simulink model "Udan_SOC"  (R2017b)
settings: Solver=FixedStepAuto  StartTime=0.0  StopTime=1000  FixedStep=0.1  RelTol=1e-3
values from neighbouring files (symbols this model uses):
  DenominatorOfIntegratorFactor = 100.0    [SOC_Stateflow.sldd]
  SOC_CalcSohLKT = 1.0    [SOC_Stateflow.sldd]
  SOC_CalcSOHTempLimit = 70.0    [SOC_Stateflow.sldd]
  SOC_CapPerCycle = 100.0    [SOC_Stateflow.sldd]
  SOC_CapTemp_HLimit = 200.0    [SOC_Stateflow.sldd]
  SOC_CapTemp_LLimit = 0.0    [SOC_Stateflow.sldd]
  Soc_ConfigInfo = 0    [SOC_Stateflow.sldd]
  SOC_DchgEndCalib = 0.0    [SOC_Stateflow.sldd]
  SOC_DiffVoltMin = 10.0    [SOC_Stateflow.sldd]
  SOC_DSOCJumpMax = 500.0    [SOC_Stateflow.sldd]
  SOC_EfficientHighLimit = 250.0    [SOC_Stateflow.sldd]
  SOC_EfficientLowLimit = 40.0    [SOC_Stateflow.sldd]
  SOC_EmptyAus = 0.0    [SOC_Stateflow.sldd]
  SOC_EnableOcv = 1.0    [SOC_Stateflow.sldd]
  SOC_END_CALIB_STATE : value not decoded    [SOC_Stateflow.sldd]
  SOC_HighRealSoc = 95.0    [SOC_Stateflow.sldd]
  SOC_LKTSohCycles = 0.0 1.0 10.0 20.0 30.0 40.0 50.0 60.0 70.0 80.0 90.0 100.0 110.0 120.0 130.0 140.0 150.0 160.0 170.0 180.0 190.0 200.0 210.0 220.0 230.0 240.0 250.0 260.0 270.0 280.0 290.0 300.0 310.0 320.0 330.0 340.0 350.0 360.0 370.0 380.0 390.0 400.0 410.0 420.0 430.0 440.0 450.0 460.0 470.0 480.0 490.0 500.0 510.0 520.0 530.0 540.0 550.0 560.0 570.0 580.0 590.0 600.0 610.0 620.0 630.0 640.0 650.0 660.0 670.0    [SOC_Stateflow.sldd]
  SOC_LKTSohTable = 1000.0 991.0 989.0 992.0 993.0 995.0 994.0 993.0 1000.0 997.0 1002.0 1000.0 992.0 1000.0 989.0 992.0 989.0 994.0 989.0 993.0 994.0 994.0 994.0 993.0 991.0 991.0 992.0 993.0 991.0 985.0 985.0 985.0 979.0 975.0 978.0 984.0 982.0 974.0 975.0 972.0 972.0 975.0 977.0 977.0 974.0 971.0 973.0 971.0 966.0 968.0 965.0 959.0 957.0 956.0 957.0 954.0 955.0 951.0 954.0 951.0 942.0 942.0 940.0 942.0 947.0 949.0    [SOC_Stateflow.sldd]
  SOC_LowRealSoc = 5.0    [SOC_Stateflow.sldd]
  SOC_NominalCap_AmS = 576000000.0    [SOC_Stateflow.sldd]
  SOC_NominalVol = 4000.0    [SOC_Stateflow.sldd]
  SOC_OCVTemp_HLimit = 106.0    [SOC_Stateflow.sldd]
  SOC_OCVTemp_LLimit = 29.0    [SOC_Stateflow.sldd]
  SOC_ShortCalibDSoc = 1.0    [SOC_Stateflow.sldd]
  SOC_SOCResolution = 10000.0    [SOC_Stateflow.sldd]
  SOC_SohCalcCapPercent = 8.0    [SOC_Stateflow.sldd]
  SOC_SohCalcHighLimit = 60.0    [SOC_Stateflow.sldd]
  SOC_SohCalcLowLimit = 10.0    [SOC_Stateflow.sldd]
  SOC_SohCalcMidLimit = 30.0    [SOC_Stateflow.sldd]
  SOC_SOHResolution = 1000.0    [SOC_Stateflow.sldd]
  SOC_State = <binary blob, 1163 chars, not shown>    [SOC_Stateflow.sldd]
  SOC_TempCap_CapBuffer : value not decoded    [SOC_Stateflow.sldd]
  SOC_TempCap_TempBuffer : value not decoded    [SOC_Stateflow.sldd]
  SocOcvCalib_ConfigInfo = 0.0    [SOC_Stateflow.sldd]
  SocOcvCalib_SocBuffer1 : value not decoded    [SOC_Stateflow.sldd]
  SocOcvCalib_TempBuffer : value not decoded    [SOC_Stateflow.sldd]
  SocOcvCalib_VoltageBuffer1 = 3300.0 3303.0 3305.0 3307.0 3310.0 3311.0 3313.0 3314.0 3316.0 3317.0 3319.0 3320.0 3322.0 3323.0 3325.0 3322.0 3323.0 3325.0 3310.0 3313.0 3315.0 3317.0 3320.0 3321.0 3323.0 3324.0 3326.0 3327.0 3329.0 3330.0 3332.0 3333.0 3335.0 3332.0 3333.0 3335.0 3320.0 3323.0 3325.0 3327.0 3330.0 3331.0 3333.0 3334.0 3336.0 3337.0 3339.0 3340.0 3342.0 3343.0 3345.0 3342.0 3343.0 3345.0 3330.0 3333.0 3335.0 3    [SOC_Stateflow.sldd]
  SOHCalibCycle = 10.0    [SOC_Stateflow.sldd]
undefined symbols (not defined in the file or in its folder): DatetimeM_GetReturnType, ParameterM_EeepParaIndexType, Soc_CumuLativeTypeType, SOC_EgthTempChgValue, Soc_EnergyBuffer, SOC_FithTempChgValue, SOC_FstSlowTempChgValue, SOC_FstTempChgValue, SOC_FthTempChgValue, SOC_MaxCap_AmS, SOC_SethTempChgValue, SOC_SixTempChgValue, SOC_SndSlowTempChgValue, SOC_SndTempChgValue, SOC_TrdSlowTempChgValue, SOC_TrdTempChgValue, SocDiagCalib_NoCalibReasonType
libraries: simulink x138, hdlsllib x24, dspindex x4
(part 5 of 10)

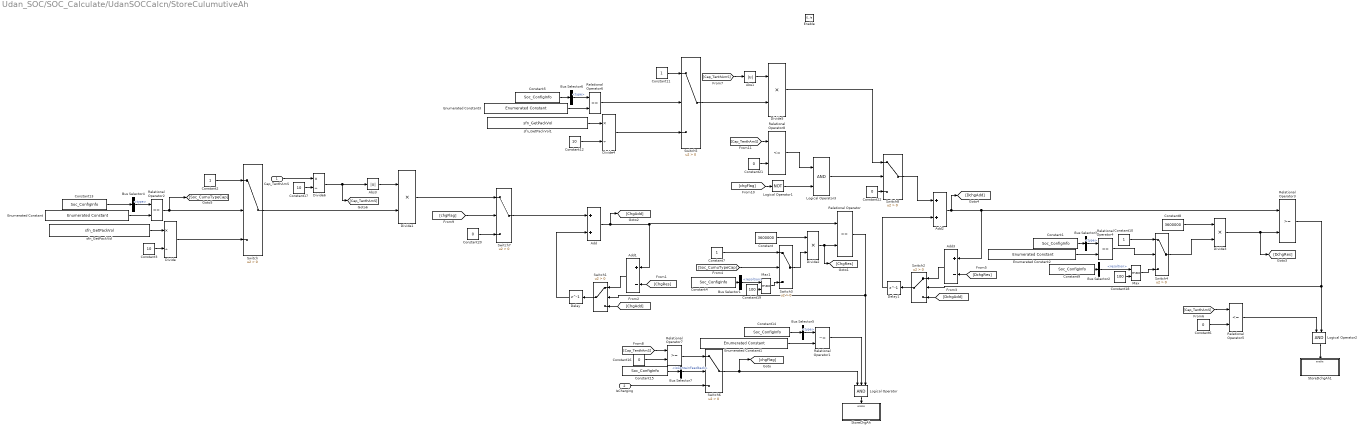
== system Udan_SOC/SOC_Calculate/UdanSOCCalcn/StoreCulumutiveAh ==
  Cap_TenthAmS : Inport
  IsCharging : Inport  Port=2
  Enable : EnablePort
  Abs1 : Abs
  Abs3 : Abs
  Add : Sum  OutDataTypeStr=uint32
  Add1 : Sum  Inputs=+-  OutDataTypeStr=int32
  Add2 : Sum  OutDataTypeStr=uint32
  Add3 : Sum  Inputs=+-  OutDataTypeStr=int32
  Bus Selector1 : BusSelector  OutputSignals=ChgCumuInfo.resoltion
  Bus Selector2 : BusSelector  OutputSignals=DchgCumuInfo.resoltion
  Bus Selector3 : BusSelector  OutputSignals=DchgCumuInfo.type
  Bus Selector4 : BusSelector  OutputSignals=ChgCumuInfo.type
  Bus Selector5 : BusSelector  OutputSignals=ChgCumuInfo.type
  Bus Selector6 : BusSelector  OutputSignals=DchgCumuInfo.type
  Bus Selector7 : BusSelector  OutputSignals=ChgCumuInfo.isContainFeedback
  Constant : Constant  Value=3600000  OutDataTypeStr=uint32
  Constant{1,4..5,9,13..15} (7 alike) : Constant  Value=Soc_ConfigInfo  OutDataTypeStr=Bus: Soc_ConfigInfoType
  Constant{2,7,10..11} (4 alike) : Constant  OutDataTypeStr=uint16
  Constant12 : Constant  Value=10  OutDataTypeStr=uint8
  Constant16 : Constant  Value=0  OutDataTypeStr=uint8
  Constant17 : Constant  Value=10  OutDataTypeStr=uint8
  Constant18 : Constant  Value=100  OutDataTypeStr=uint16
  Constant19 : Constant  Value=100  OutDataTypeStr=uint16
  Constant20 : Constant  Value=0  OutDataTypeStr=uint32
  Constant21 : Constant  Value=0  OutDataTypeStr=int8
  Constant22 : Constant  Value=0  OutDataTypeStr=uint32
  Constant3 : Constant  Value=10  OutDataTypeStr=uint8
  Constant6 : Constant  Value=0  OutDataTypeStr=uint8
  Constant8 : Constant  Value=3600000  OutDataTypeStr=uint32
  Delay : Delay  DelayLength=1  InitialCondition=0
  Delay1 : Delay  DelayLength=1  InitialCondition=0
  Divide : Product  Inputs=*/  OutDataTypeStr=uint16
  Divide{1..3,5} (4 alike) : Product  Inputs=**  OutDataTypeStr=uint32
  Divide4 : Product  Inputs=*/  OutDataTypeStr=uint16
  Divide6 : Product  Inputs=*/  OutDataTypeStr=int32
  Enumerated Constant : simulink/Sources/Enumerated Constant  OutDataTypeStr=Enum: Soc_CumuLativeTypeType  Value=Soc_CumuLativeTypeType.Soc_CumuTypeCap  SampleTime=inf
      settings: SourceProductName=Simulink
  Enumerated Constant1 : simulink/Sources/Enumerated Constant  OutDataTypeStr=Enum: Soc_CumuLativeTypeType  Value=Soc_CumuLativeTypeType.Soc_CumuTypeNone  SampleTime=inf
      settings: SourceProductName=Simulink
  Enumerated Constant2 : simulink/Sources/Enumerated Constant  OutDataTypeStr=Enum: Soc_CumuLativeTypeType  Value=Soc_CumuLativeTypeType.Soc_CumuTypeCap  SampleTime=inf
      settings: SourceProductName=Simulink
  Enumerated Constant3 : simulink/Sources/Enumerated Constant  OutDataTypeStr=Enum: Soc_CumuLativeTypeType  Value=Soc_CumuLativeTypeType.Soc_CumuTypeCap  SampleTime=inf
      settings: SourceProductName=Simulink
  Logical Operator : Logic  Inputs=3  AllPortsSameDT=off  OutDataTypeStr=boolean
  Logical Operator1 : Logic  Operator=NOT  AllPortsSameDT=off  OutDataTypeStr=boolean
  Logical Operator2 : Logic  AllPortsSameDT=off  OutDataTypeStr=boolean
  Logical Operator3 : Logic  AllPortsSameDT=off  OutDataTypeStr=boolean
  Max : MinMax  Function=max  Inputs=2
  Max1 : MinMax  Function=max  Inputs=2
  Relational Operator : RelationalOperator  OutDataTypeStr=boolean  RndMeth=Simplest
  Relational Operator1 : RelationalOperator  Operator=~=  OutDataTypeStr=boolean  RndMeth=Simplest
  Relational Operator2 : RelationalOperator  Operator===  OutDataTypeStr=boolean  RndMeth=Simplest
  Relational Operator3 : RelationalOperator  OutDataTypeStr=boolean  RndMeth=Simplest
  Relational Operator4 : RelationalOperator  Operator===  OutDataTypeStr=boolean  RndMeth=Simplest
  Relational Operator5 : RelationalOperator  Operator=<=  OutDataTypeStr=boolean  RndMeth=Simplest
  Relational Operator6 : RelationalOperator  Operator===  OutDataTypeStr=boolean  RndMeth=Simplest
  Relational Operator7 : RelationalOperator  OutDataTypeStr=boolean  RndMeth=Simplest
  Relational Operator8 : RelationalOperator  Operator=<=  OutDataTypeStr=boolean  RndMeth=Simplest
  StoreChgAh : Subsystem  TreatAsAtomicUnit=on
  StoreDchgAh1 : Subsystem  TreatAsAtomicUnit=on
  Switch{,1..2,5..8} (7 alike) : Switch  Criteria=u2 > Threshold
  Switch3 : Switch  Criteria=u2 > Threshold  OutDataTypeStr=uint16
  Switch4 : Switch  Criteria=u2 > Threshold  OutDataTypeStr=uint16
  sfn_GetPackVol : S-Function  FunctionName=sfn_GetPackVol  SFunctionDeploymentMode=off  EnableBusSupport=off  mask(Legacy Function){SFunctionSpec=uint16 y1=Statistic_GetBcu100mvTotalVoltage(void), ShowSpec=on}
      mask prompts: ShowSpec "Display function specification"
      mask help:
      | This block allows you to call the legacy functions specified by the following Legacy Code Tool definition:
      | def.SFunctionName = 'sfn_GetPackVol';
      | def.OutputFcnSpec = 'uint16 y1=Statistic_GetBcu100mvTotalVoltage(void)';
      | def.HeaderFiles = {'Statistic.h'};
      mask Help: <p>This block was generated automatically by the Legacy Code Tool. For detailed help on this tool, call<a href="matlab:legacy_code('help')"> legacy_code('help')</a>.</p>
      mask Callback ShowSpec:
      | if strcmp(get_param(gcbh, 'ShowSpec'), 'on')
      |   set_param(gcbh, 'MaskDisplay', sprintf('fprintf(''%s'');', get_param(gcbh, 'SFunctionSpec')));
      | else
      |   set_param(gcbh, 'MaskDisplay', sprintf('fprintf(''%s'');', get_param(gcbh, 'FunctionName')));
      | end
      mask Display: fprintf('uint16 y1=Statistic_GetBcu100mvTotalVoltage(void)');
  sfn_GetPackVol1 : S-Function  FunctionName=sfn_GetPackVol  SFunctionDeploymentMode=off  EnableBusSupport=off  mask(Legacy Function){SFunctionSpec=uint16 y1=Statistic_GetBcu100mvTotalVoltage(void), ShowSpec=on}
      mask prompts: ShowSpec "Display function specification"
      mask help:
      | This block allows you to call the legacy functions specified by the following Legacy Code Tool definition:
      | def.SFunctionName = 'sfn_GetPackVol';
      | def.OutputFcnSpec = 'uint16 y1=Statistic_GetBcu100mvTotalVoltage(void)';
      | def.HeaderFiles = {'Statistic.h'};
      mask Help: <p>This block was generated automatically by the Legacy Code Tool. For detailed help on this tool, call<a href="matlab:legacy_code('help')"> legacy_code('help')</a>.</p>
      mask Callback ShowSpec:
      | if strcmp(get_param(gcbh, 'ShowSpec'), 'on')
      |   set_param(gcbh, 'MaskDisplay', sprintf('fprintf(''%s'');', get_param(gcbh, 'SFunctionSpec')));
      | else
      |   set_param(gcbh, 'MaskDisplay', sprintf('fprintf(''%s'');', get_param(gcbh, 'FunctionName')));
      | end
      mask Display: fprintf('uint16 y1=Statistic_GetBcu100mvTotalVoltage(void)');
  wires:
  Abs3/1 -> Divide1/1
  Switch7/1 -> Add/1
  Bus Selector3/1 -> Relational Operator4/1  "<type>"
  Constant1/1 -> Bus Selector3/1
  Enumerated Constant2/1 -> Relational Operator4/2
  Constant14/1 -> Bus Selector5/1
  Relational Operator1/1 -> Logical Operator/2
  Enumerated Constant1/1 -> Relational Operator1/2
  Bus Selector5/1 -> Relational Operator1/1  "<type>"
  Add2/1 -> [DchgAdd], Add3/1, Relational Operator3/1
  Delay1/1 -> Add2/2
  [DchgRes] -> Add3/2
  Switch2/1 -> Delay1/1
  [DchgAdd] -> Switch2/3
  Add3/1 -> Switch2/1
  Delay/1 -> Add/2
  [ChgAdd] -> Switch1/3
  Add1/1 -> Switch1/1
  [ChgRes] -> Add1/2
  Relational Operator/1 -> Logical Operator/3, Switch1/2
  Relational Operator3/1 -> Logical Operator2/2, Switch2/2
  Divide3/1 -> Relational Operator3/2, [DchgRes]
  Divide2/1 -> [ChgRes], Relational Operator/2
  Constant4/1 -> Bus Selector1/1
  Bus Selector1/1 -> Max1/1  "<resoltion>"
  IsCharging/1 -> Switch6/3
  Switch/1 -> Divide1/2
  Divide6/1 -> [Cap_TenthAmS], Abs3/1
  Divide/1 -> Switch/3
  Constant3/1 -> Divide/2
  sfn_GetPackVol/1 -> Divide/1
  Constant2/1 -> Switch/1
  Relational Operator2/1 -> Switch/2, [Soc_CumuTypeCap]
  Enumerated Constant/1 -> Relational Operator2/2
  Constant13/1 -> Bus Selector4/1
  Bus Selector4/1 -> Relational Operator2/1  "<type>"
  Logical Operator2/1 -> StoreDchgAh1/Enable
  Logical Operator/1 -> StoreChgAh/Enable
  Constant/1 -> Divide2/1
  Add/1 -> Add1/1, Relational Operator/1, [ChgAdd]
  Switch1/1 -> Delay/1
  [Soc_CumuTypeCap] -> Switch3/2
  Constant7/1 -> Switch3/1
  Switch3/1 -> Divide2/2
  Relational Operator5/1 -> Logical Operator2/1
  [Cap_TenthAmS] -> Relational Operator5/1
  Constant6/1 -> Relational Operator5/2
  Switch4/1 -> Divide3/2
  Bus Selector2/1 -> Max/1  "<resoltion>"
  Constant9/1 -> Bus Selector2/1
  Constant8/1 -> Divide3/1
  Relational Operator4/1 -> Switch4/2
  Constant10/1 -> Switch4/1
  Constant11/1 -> Switch5/1
  Relational Operator6/1 -> Switch5/2
  Constant5/1 -> Bus Selector6/1
  Enumerated Constant3/1 -> Relational Operator6/2
  Bus Selector6/1 -> Relational Operator6/1  "<type>"
  Constant12/1 -> Divide4/2
  Divide4/1 -> Switch5/3
  sfn_GetPackVol1/1 -> Divide4/1
  [Cap_TenthAmS] -> Abs1/1
  Switch5/1 -> Divide5/2
  Divide5/1 -> Switch8/1
  Abs1/1 -> Divide5/1
  Constant15/1 -> Bus Selector7/1
  Constant16/1 -> Relational Operator7/2
  [Cap_TenthAmS] -> Relational Operator7/1
  Bus Selector7/1 -> Switch6/2  "<isContainFeedback>"
  Relational Operator7/1 -> Switch6/1
  Switch6/1 -> [chgFlag], Logical Operator/1
  Cap_TenthAmS/1 -> Divide6/1
  Constant17/1 -> Divide6/2
  Constant18/1 -> Max/2
  Max/1 -> Switch4/3
  Constant19/1 -> Max1/2
  Max1/1 -> Switch3/3
  [chgFlag] -> Switch7/2
  Divide1/1 -> Switch7/1
  Constant20/1 -> Switch7/3
  [chgFlag] -> Logical Operator1/1
  [Cap_TenthAmS] -> Relational Operator8/1
  Constant21/1 -> Relational Operator8/2
  Relational Operator8/1 -> Logical Operator3/1
  Logical Operator1/1 -> Logical Operator3/2
  Logical Operator3/1 -> Switch8/2
  Constant22/1 -> Switch8/3
  Switch8/1 -> Add2/1

== system Udan_SOC/SOC_Calculate/UdanSOCCalcn/StoreDSOC ==
  LastCap : Inport
  SocCalibFlag : Inport  Port=2  OutDataTypeStr=uint8  PortDimensions=[1]
  OcvCmd : Inport  Port=3
  Abs : Abs
  Bus Selector : BusSelector  OutputSignals=soc
  Constant1 : Constant  OutDataTypeStr=uint8
  Constant6 : Constant  Value=50  OutDataTypeStr=uint8
  Delay1 : Delay  DelayLength=1  InitialCondition=0
  Logical Operator : Logic  AllPortsSameDT=off  OutDataTypeStr=boolean
  Logical Operator1 : Logic  Operator=OR  Inputs=3  AllPortsSameDT=off  OutDataTypeStr=boolean
  Relational Operator1 : RelationalOperator  OutDataTypeStr=boolean  RndMeth=Simplest
  Relational Operator3 : RelationalOperator  OutDataTypeStr=boolean  RndMeth=Simplest
  Subtract : Sum  Inputs=+-  AccumDataTypeStr=int32  OutDataTypeStr=int32
  Switch : Switch  Criteria=u2 > Threshold
  WriteLeftCap : Subsystem  TreatAsAtomicUnit=on
  wires:
  Bus Selector/1 -> Relational Operator1/1, Switch/1, WriteLeftCap/1(DSOC), Subtract/2  "<soc>"
  Relational Operator3/1 -> Logical Operator1/3, Switch/2
  Switch/1 -> Delay1/1
  Delay1/1 -> Switch/3, [WritedCap]
  Abs/1 -> Relational Operator3/1
  Constant6/1 -> Relational Operator3/2
  Subtract/1 -> Abs/1
  [WritedCap] -> Subtract/1
  LastCap/1 -> Bus Selector/1
  Logical Operator/1 -> WriteLeftCap/Enable
  Constant1/1 -> Relational Operator1/2
  Relational Operator1/1 -> Logical Operator/1
  Logical Operator1/1 -> Logical Operator/2
  SocCalibFlag/1 -> Logical Operator1/2
  OcvCmd/1 -> Logical Operator1/1

== system Udan_SOC/SOC_Calculate/UdanSOCCalcn/StoreLeftCap ==
  LastCap : Inport
  OcvCmd : Inport  Port=2
  SocCalibFlag : Inport  Port=3  OutDataTypeStr=uint8  PortDimensions=[1]
  Constant : Constant  Value=SOC_SOCResolution
  Constant1 : Constant  Value=SOC_NominalCap_AmS
  Constant4 : Constant  Value=SOC_NominalCap_AmS
  Constant5 : Constant  Value=1000  OutDataTypeStr=uint32
  Constant6 : Constant  Value=8  OutDataTypeStr=uint32
  Delay1 : Delay  DelayLength=1  InitialCondition=0
  Divide : Product  Inputs=*/*
  Divide1 : Product  Inputs=*/  OutDataTypeStr=uint32
  Logical Operator : Logic  AllPortsSameDT=off  OutDataTypeStr=boolean
  Logical Operator1 : Logic  Operator=OR  Inputs=3  AllPortsSameDT=off  OutDataTypeStr=boolean
  Logical Operator2 : Logic  Operator=NOT  AllPortsSameDT=off  OutDataTypeStr=boolean
  Relational Operator : RelationalOperator  OutDataTypeStr=boolean  RndMeth=Simplest
  Relational Operator1 : RelationalOperator  OutDataTypeStr=boolean  RndMeth=Simplest
  Relational Operator3 : RelationalOperator  OutDataTypeStr=boolean  RndMeth=Simplest
  Subtract : Sum  Inputs=+-  AccumDataTypeStr=uint32  OutDataTypeStr=uint32
  Switch : Switch  Criteria=u2 > Threshold
  Switch1 : Switch  Criteria=u2 > Threshold
  Switch2 : Switch  Criteria=u2 > Threshold
  WriteLeftCap : Subsystem  TreatAsAtomicUnit=on
  wires:
  LastCap/1 -> Switch2/3, Switch1/3, Relational Operator/2, WriteLeftCap/1(cap), Switch/1, Relational Operator1/1
  Relational Operator3/1 -> Logical Operator1/3, Switch/2
  Switch/1 -> Delay1/1
  Delay1/1 -> Switch/3, [WritedCap]
  Subtract/1 -> Relational Operator3/1
  Divide/1 -> Relational Operator3/2
  Constant6/1 -> Divide/3
  Constant5/1 -> Divide/2
  Constant4/1 -> Divide/1
  [WritedCap] -> Relational Operator/1, Switch2/1, Switch1/1
  Constant1/1 -> Divide1/1
  Constant/1 -> Divide1/2
  Divide1/1 -> Relational Operator1/2
  Relational Operator1/1 -> Logical Operator/1
  Logical Operator/1 -> WriteLeftCap/Enable
  Logical Operator1/1 -> Logical Operator/2
  SocCalibFlag/1 -> Logical Operator1/1
  Relational Operator/1 -> Switch1/2, Logical Operator2/1
  Switch1/1 -> Subtract/1
  Logical Operator2/1 -> Switch2/2
  Switch2/1 -> Subtract/2
  OcvCmd/1 -> Logical Operator1/2

== system Udan_SOC/SOC_Calculate/UdanSOCCalcn/StoreSOC ==
  CurrentAmS : Inport
  IsCharging : Inport  Port=2
  Constant : Constant  Value=0  OutDataTypeStr=uint8
  Constant1 : Constant  Value=0  OutDataTypeStr=uint8
  Logical Operator : Logic  Operator=OR  AllPortsSameDT=off  OutDataTypeStr=boolean
  Logical Operator1 : Logic  AllPortsSameDT=off  OutDataTypeStr=boolean
  Logical Operator2 : Logic  Operator=NOT  AllPortsSameDT=off  OutDataTypeStr=boolean
  Relational Operator : RelationalOperator  Operator=<=  OutDataTypeStr=boolean  RndMeth=Simplest
  Relational Operator1 : RelationalOperator  Operator=>  OutDataTypeStr=boolean  RndMeth=Simplest
  Subsystem : Subsystem
  Subsystem1 : Subsystem
  wires:
  Constant/1 -> Relational Operator/2
  Relational Operator/1 -> Logical Operator/1
  Logical Operator/1 -> Subsystem/Enable
  IsCharging/1 -> [IsCharging], Logical Operator/2
  CurrentAmS/1 -> Relational Operator/1, Subsystem/1(CurrentAmS), Subsystem1/1(CurrentAmS), Relational Operator1/1
  Constant1/1 -> Relational Operator1/2
  Relational Operator1/1 -> Logical Operator1/1
  [IsCharging] -> Logical Operator2/1
  Logical Operator2/1 -> Logical Operator1/2
  Logical Operator1/1 -> Subsystem1/Enable

== system Udan_SOC/SOC_Calculate/UdanSOCCalcn/StoreTSOC ==
  LastCap : Inport
  Abs : Abs
  Bus Selector : BusSelector  OutputSignals=soc
  Constant1 : Constant  OutDataTypeStr=uint8
  Constant6 : Constant  Value=100  OutDataTypeStr=uint8
  Delay1 : Delay  DelayLength=1  InitialCondition=0
  Logical Operator : Logic  AllPortsSameDT=off  OutDataTypeStr=boolean
  Logical Operator1 : Logic  Operator=OR  Inputs=1  AllPortsSameDT=off  OutDataTypeStr=boolean
  Relational Operator1 : RelationalOperator  OutDataTypeStr=boolean  RndMeth=Simplest
  Relational Operator3 : RelationalOperator  OutDataTypeStr=boolean  RndMeth=Simplest
  Subtract : Sum  Inputs=+-  AccumDataTypeStr=int32  OutDataTypeStr=int32
  Switch : Switch  Criteria=u2 > Threshold
  WriteLeftCap : Subsystem  TreatAsAtomicUnit=on
  wires:
  Bus Selector/1 -> Relational Operator1/1, Switch/1, WriteLeftCap/1(DSOC), Subtract/2  "<soc>"
  Relational Operator3/1 -> Logical Operator1/1, Switch/2
  Switch/1 -> Delay1/1
  Delay1/1 -> Switch/3, [WritedCap]
  Abs/1 -> Relational Operator3/1
  Constant6/1 -> Relational Operator3/2
  Subtract/1 -> Abs/1
  [WritedCap] -> Subtract/1
  LastCap/1 -> Bus Selector/1
  Logical Operator/1 -> WriteLeftCap/Enable
  Constant1/1 -> Relational Operator1/2
  Relational Operator1/1 -> Logical Operator/1
  Logical Operator1/1 -> Logical Operator/2

== system Udan_SOC/SOC_Calculate/UdanSOCCalcn/Subsystem1 ==
  HighIndex : Inport
  LowIndex : Inport  Port=2
  DefaultValue : Inport  Port=3
  Constant1 : Constant  Value=0  OutDataTypeStr=uint8
  Constant2 : Constant  Value=0  OutDataTypeStr=uint8
  Logical Operator : Logic  AllPortsSameDT=off  OutDataTypeStr=boolean
  Logical Operator1 : Logic  Operator=NOT  AllPortsSameDT=off  OutDataTypeStr=boolean
  Relational Operator : RelationalOperator  Operator===  OutDataTypeStr=boolean  RndMeth=Simplest
  Relational Operator1 : RelationalOperator  Operator===  OutDataTypeStr=boolean  RndMeth=Simplest
  S-Function : S-Function  FunctionName=sfn_NVMRead  SFunctionDeploymentMode=off  EnableBusSupport=off
  S-Function1 : S-Function  FunctionName=sfn_NVMRead  SFunctionDeploymentMode=off  EnableBusSupport=off
  Subsystem : Subsystem
  Switch : Switch  Criteria=u2 > Threshold
  EeepRead32 : Outport
  wires:
  DefaultValue/1 -> Switch/1
  [ReadLowOk] -> Logical Operator/1
  S-Function/2 -> Subsystem/1(HighIndex)
  S-Function/1 -> Relational Operator/1
  S-Function1/2 -> Subsystem/2(LowIndex)
  HighIndex/1 -> S-Function/1
  Constant1/1 -> Relational Operator/2
  Constant2/1 -> Relational Operator1/2
  LowIndex/1 -> S-Function1/1
  Relational Operator/1 -> Logical Operator/2
  Logical Operator/1 -> Logical Operator1/1, Subsystem/Enable
  Relational Operator1/1 -> [ReadLowOk]
  S-Function1/1 -> Relational Operator1/1
  Subsystem/1(soc) -> Switch/3
  Logical Operator1/1 -> Switch/2
  Switch/1 -> EeepRead32/1

== system Udan_SOC/SOC_Calculate/UdanSOCCalcn/WriteOCVTime ==
  RTCTimeOut : Inport
  OCVCmd : Inport  Port=2
  RtcTime : Inport  Port=3
  function : TriggerPort  TriggerType=function-call  VariantControl=Variant
  Constant : Constant  Value=0  OutDataTypeStr=boolean
  Data Store Write : DataStoreWrite  DataStoreName=LargeCurrentFlag
  Enumerated Constant : simulink/Sources/Enumerated Constant  OutDataTypeStr=Enum: ParameterM_EeepParaIndexType  Value=ParameterM_EeepParaIndexType.PARAMETERM_EEEP_OCVSOC_TIME_HIGH_INDEX  SampleTime=inf
      settings: SourceProductName=Simulink
  Enumerated Constant1 : simulink/Sources/Enumerated Constant  OutDataTypeStr=Enum: ParameterM_EeepParaIndexType  Value=ParameterM_EeepParaIndexType.PARAMETERM_EEEP_OCVSOC_TIME_LOW_INDEX  SampleTime=inf
      settings: SourceProductName=Simulink
  Enumerated Constant2 : simulink/Sources/Enumerated Constant  OutDataTypeStr=Enum: SOC_State  Value=SOC_State.SOC_STATE_DCHGSOH  SampleTime=inf
      settings: SourceProductName=Simulink
  Enumerated Constant6 : simulink/Sources/Enumerated Constant  OutDataTypeStr=Enum: SOC_State  Value=SOC_State.SOC_STATE_OCV_LONG  SampleTime=inf
      settings: SourceProductName=Simulink
  Enumerated Constant7 : simulink/Sources/Enumerated Constant  OutDataTypeStr=Enum: SOC_State  Value=SOC_State.SOC_STATE_OCV  SampleTime=inf
      settings: SourceProductName=Simulink
  Logical Operator : Logic  Operator=OR  Inputs=3  AllPortsSameDT=off  OutDataTypeStr=boolean
  Relational Operator1 : RelationalOperator  Operator===  OutDataTypeStr=boolean  RndMeth=Simplest
  Relational Operator10 : RelationalOperator  Operator===  OutDataTypeStr=boolean  RndMeth=Simplest
  Relational Operator11 : RelationalOperator  Operator===  OutDataTypeStr=boolean  RndMeth=Simplest
  Subsystem : Subsystem  mask(EeepWrite_uint32){}
      mask help: EeepWrite_uint32
  Switch8 : Switch  Criteria=u2 > Threshold
  Terminator : Terminator
  SOC_RTCTime : Outport
  wires:
  RtcTime/1 -> Switch8/1
  Enumerated Constant1/1 -> Subsystem/3(LowIndex)
  Enumerated Constant/1 -> Subsystem/2(HighIndex)
  Constant/1 -> Data Store Write/1
  RTCTimeOut/1 -> Switch8/3
  Switch8/1 -> SOC_RTCTime/1, Subsystem/1(data)
  Enumerated Constant6/1 -> Relational Operator11/2
  Enumerated Constant7/1 -> Relational Operator10/2
  Enumerated Constant2/1 -> Relational Operator1/2
  OCVCmd/1 -> Relational Operator1/1, Relational Operator11/1, Relational Operator10/1
  Relational Operator11/1 -> Logical Operator/2
  Relational Operator10/1 -> Logical Operator/1
  Relational Operator1/1 -> Logical Operator/3
  Logical Operator/1 -> Switch8/2
  Subsystem/1(WriteResult) -> Terminator/1

== system Udan_SOC/SOC_Calculate/UdanSOCCalcn/WriteSOH ==
  SOH : Inport
  Enable : EnablePort
  Data Type Conversion : DataTypeConversion  OutDataTypeStr=uint16
  Enabled Subsystem : Subsystem  TreatAsAtomicUnit=on
  Enabled Subsystem1 : Subsystem  TreatAsAtomicUnit=on
  Enabled Subsystem2 : Subsystem  TreatAsAtomicUnit=on
  Enabled Subsystem3 : Subsystem  TreatAsAtomicUnit=on
  Enabled Subsystem4 : Subsystem  TreatAsAtomicUnit=on
  Enabled Subsystem5 : Subsystem  TreatAsAtomicUnit=on
  Enabled Subsystem6 : Subsystem  TreatAsAtomicUnit=on
  Enabled Subsystem7 : Subsystem  TreatAsAtomicUnit=on
  Enumerated Constant2 : simulink/Sources/Enumerated Constant  OutDataTypeStr=Enum: ParameterM_EeepParaIndexType  Value=ParameterM_EeepParaIndexType.PARAMETERM_EEEP_SOH_INDEX  SampleTime=inf
      settings: SourceProductName=Simulink
  Logical Operator{,2,4,6} (4 alike) : Logic  Operator=NOT  AllPortsSameDT=off  OutDataTypeStr=boolean
  Logical Operator{1,3,5,7} (4 alike) : Logic  Operator=OR  AllPortsSameDT=off  OutDataTypeStr=boolean
  Logical Operator{8..13} (6 alike) : Logic  AllPortsSameDT=off  OutDataTypeStr=boolean
  S-Function : S-Function  FunctionName=sfn_NVMWrite  SFunctionDeploymentMode=off  EnableBusSupport=off
  Terminator : Terminator
  wires:
  Enumerated Constant2/1 -> [index], S-Function/1
  SOH/1 -> Data Type Conversion/1
  S-Function/1 -> Logical Operator1/1, Logical Operator/1
  Data Type Conversion/1 -> [data], S-Function/2
  [index] -> Enabled Subsystem/1(index)
  [data] -> Enabled Subsystem/2(data)
  [index] -> Enabled Subsystem1/1(index)
  [data] -> Enabled Subsystem1/2(data)
  [index] -> Enabled Subsystem2/1(index)
  [data] -> Enabled Subsystem2/2(data)
  [index] -> Enabled Subsystem3/1(index)
  [data] -> Enabled Subsystem3/2(data)
  Enabled Subsystem3/1(EeepWriteFailure) -> Terminator/1
  Logical Operator/1 -> Enabled Subsystem4/Enable
  [data] -> Enabled Subsystem4/2(data)
  [index] -> Enabled Subsystem4/1(index)
  Logical Operator1/1 -> Logical Operator8/1, Logical Operator9/2, Enabled Subsystem/Enable
  Enabled Subsystem4/1(EeepWriteFailure) -> Logical Operator1/2
  [index] -> Enabled Subsystem5/1(index)
  Logical Operator2/1 -> Logical Operator8/2
  Enabled Subsystem/1(EeepWriteFailure) -> Logical Operator3/1, Logical Operator2/1
  Logical Operator3/1 -> Logical Operator9/1
  Enabled Subsystem5/1(EeepWriteFailure) -> Logical Operator3/2
  [data] -> Enabled Subsystem5/2(data)
  [data] -> Enabled Subsystem6/2(data)
  Logical Operator4/1 -> Logical Operator10/2
  [index] -> Enabled Subsystem6/1(index)
  Enabled Subsystem1/1(EeepWriteFailure) -> Logical Operator5/1, Logical Operator4/1
  Enabled Subsystem6/1(EeepWriteFailure) -> Logical Operator5/2
  Logical Operator5/1 -> Logical Operator11/1
  Logical Operator6/1 -> Logical Operator12/2
  [index] -> Enabled Subsystem7/1(index)
  [data] -> Enabled Subsystem7/2(data)
  Logical Operator7/1 -> Logical Operator13/1
  Enabled Subsystem2/1(EeepWriteFailure) -> Logical Operator7/1, Logical Operator6/1
  Enabled Subsystem7/1(EeepWriteFailure) -> Logical Operator7/2
  Logical Operator8/1 -> Enabled Subsystem5/Enable
  Logical Operator9/1 -> Logical Operator10/1, Logical Operator11/2, Enabled Subsystem1/Enable
  Logical Operator11/1 -> Logical Operator12/1, Logical Operator13/2, Enabled Subsystem2/Enable
  Logical Operator10/1 -> Enabled Subsystem6/Enable
  Logical Operator13/1 -> Enabled Subsystem3/Enable
  Logical Operator12/1 -> Enabled Subsystem7/Enable

== system Udan_SOC/SOC_Calculate/UdanSOCCalcn/CalcChgSOH/Subsystem ==
  SOC_LeftCap : Inport
  TotalCap : Inport  Port=2
  LookUpLeftCap : Inport  Port=3
  SOHIn : Inport  Port=4
  Enable : EnablePort
  Add : Sum  Inputs=+-  AccumDataTypeStr=uint32  OutDataTypeStr=uint32
  Chart2 : Stateflow chart  TreatAsAtomicUnit=on
  Constant1 : Constant  Value=1200  OutDataTypeStr=uint16
  Constant2 : Constant  Value=800  OutDataTypeStr=uint16
  Constant25 : Constant  Value=SOC_NominalCap_AmS
  Constant{3,5,7,42} (4 alike) : Constant  Value=SOC_SOHResolution  OutDataTypeStr=uint16
  Constant31 : Constant  Value=SOC_NominalCap_AmS
  Constant4 : Constant  Value=SOC_SohCalcHighLimit
  Constant43 : Constant  Value=SOC_TempCap_CapBuffer
  Constant6 : Constant  Value=SOC_SohCalcLowLimit
  Constant8 : Constant  Value=SOC_SohCalcMidLimit
  Divide : Product  Inputs=*/  OutDataTypeStr=uint32
  Divide1 : Product  Inputs=*/  OutDataTypeStr=uint32
  Divide16 : Product  Inputs=*/*  OutDataTypeStr=uint32
  Divide2 : Product  Inputs=*/*  OutDataTypeStr=uint32
  Divide3 : Product  Inputs=*/*  OutDataTypeStr=uint32
  MinMax : MinMax  Function=max
  MinMax1 : MinMax  Function=max  Inputs=2
  Saturation Dynamic : simulink/Discontinuities/Saturation Dynamic  OutMin=[]  OutMax=[]  OutDataTypeStr=Inherit: Same as second input  OutDataType=fixdt(1, 16)  OutScaling=2^-10  DoSatur=off
  Terminator : Terminator
  Terminator1 : Terminator
  SohOut : Outport
  wires:
  SOHIn/1 -> [SOHIn], Divide3/3
  Saturation Dynamic/1 -> Chart2/1(CalcSOH)
  TotalCap/1 -> Terminator1/1  "TotalCap"
  Constant2/1 -> Saturation Dynamic/3
  Chart2/1(SOHWriteResult) -> Terminator/1
  Chart2/2(SohOut) -> SohOut/1
  Divide/1 -> Saturation Dynamic/2  "CalcnChgSOH"
  Constant1/1 -> Saturation Dynamic/1
  Divide1/1 -> Divide/2
  Constant7/1 -> Divide1/2
  SOC_LeftCap/1 -> Divide3/1
  LookUpLeftCap/1 -> Add/2  "LookTableCap"
  Add/1 -> Divide1/1  "DeltaLeftCap"
  Constant3/1 -> Divide2/2
  Divide2/1 -> Add/1
  Constant5/1 -> Divide3/2
  Divide3/1 -> Divide/1
  [SOHIn] -> Divide2/3
  [SOHIn] -> Chart2/5(EEEPSOH)
  Constant4/1 -> Chart2/2(MaxDiff)
  Constant8/1 -> Chart2/3(MaxCal)
  Constant6/1 -> Chart2/4(MaxCal1)
  MinMax1/1 -> Divide2/1
  Constant42/1 -> Divide16/2
  Constant43/1 -> MinMax/1
  MinMax/1 -> Divide16/3
  Divide16/1 -> MinMax1/1
  Constant25/1 -> MinMax1/2
  Constant31/1 -> Divide16/1

== system Udan_SOC/SOC_Calculate/UdanSOCCalcn/CalcChgSOH/Subsystem1 ==
  HighIndex : Inport
  LowIndex : Inport  Port=2
  DefaultValue : Inport  Port=3
  Constant1 : Constant  Value=0  OutDataTypeStr=uint8
  Constant2 : Constant  Value=0  OutDataTypeStr=uint8
  Logical Operator : Logic  AllPortsSameDT=off  OutDataTypeStr=boolean
  Logical Operator1 : Logic  Operator=NOT  AllPortsSameDT=off  OutDataTypeStr=boolean
  Relational Operator : RelationalOperator  Operator===  OutDataTypeStr=boolean  RndMeth=Simplest
  Relational Operator1 : RelationalOperator  Operator===  OutDataTypeStr=boolean  RndMeth=Simplest
  S-Function : S-Function  FunctionName=sfn_NVMRead  SFunctionDeploymentMode=off  EnableBusSupport=off
  S-Function1 : S-Function  FunctionName=sfn_NVMRead  SFunctionDeploymentMode=off  EnableBusSupport=off
  Subsystem : Subsystem
  Switch : Switch  Criteria=u2 > Threshold
  EeepRead32 : Outport
  wires:
  DefaultValue/1 -> Switch/1
  [ReadLowOk] -> Logical Operator/1
  S-Function/2 -> Subsystem/1(HighIndex)
  S-Function/1 -> Relational Operator/1
  S-Function1/2 -> Subsystem/2(LowIndex)
  HighIndex/1 -> S-Function/1
  Constant1/1 -> Relational Operator/2
  Constant2/1 -> Relational Operator1/2
  LowIndex/1 -> S-Function1/1
  Relational Operator/1 -> Logical Operator/2
  Logical Operator/1 -> Logical Operator1/1, Subsystem/Enable
  Relational Operator1/1 -> [ReadLowOk]
  S-Function1/1 -> Relational Operator1/1
  Subsystem/1(soc) -> Switch/3
  Logical Operator1/1 -> Switch/2
  Switch/1 -> EeepRead32/1

== system Udan_SOC/SOC_Calculate/UdanSOCCalcn/CalcDchgSOH/Subsystem ==
  SOC_LeftCap0 : Inport
  SOC_LeftCap2 : Inport  Port=2
  SOHIn : Inport  Port=3
  WOCalibAh : Inport  Port=4
  Enable : EnablePort
  Chart1 : Stateflow chart  TreatAsAtomicUnit=on
  Constant1 : Constant  Value=1200  OutDataTypeStr=uint16
  Constant10 : Constant  Value=65535  OutDataTypeStr=uint16
  Constant2 : Constant  Value=800  OutDataTypeStr=uint16
  Constant3 : Constant  Value=SOC_SohCalcHighLimit
  Constant31 : Constant  Value=SOC_NominalCap_AmS
  Constant4 : Constant  Value=1000  OutDataTypeStr=uint16
  Constant5 : Constant  Value=SOC_SohCalcLowLimit
  Constant6 : Constant  Value=SOC_SohCalcMidLimit
  Constant7 : Constant  Value=SOC_SOCResolution  OutDataTypeStr=uint16
  Constant8 : Constant  Value=1000  OutDataTypeStr=uint16
  Constant9 : Constant  Value=1000  OutDataTypeStr=uint16
  DchgPower1 : simulink/Sources/Enumerated Constant  OutDataTypeStr=Enum: ParameterM_EeepParaIndexType  Value=ParameterM_EeepParaIndexType.PARAMETERM_EEEP_SOH_Full_INDEX  SampleTime=inf
      settings: SourceProductName=Simulink
  Divide : Product  Inputs=**  OutDataTypeStr=uint32
  Divide1 : Product  Inputs=*/  OutDataTypeStr=uint32
  Divide2 : Product  Inputs=*/  OutDataTypeStr=uint32
  Divide3 : Product  Inputs=*/  OutDataTypeStr=uint32
  Divide4 : Product  Inputs=*/*  OutDataTypeStr=uint32
  Relational Operator : RelationalOperator  Operator=~=  OutDataTypeStr=boolean  RndMeth=Simplest
  S-Function1 : S-Function  FunctionName=sfn_NVMWrite  SFunctionDeploymentMode=off  EnableBusSupport=off
  Saturation Dynamic : simulink/Discontinuities/Saturation Dynamic  OutMin=[]  OutMax=[]  OutDataTypeStr=Inherit: Same as second input  OutDataType=fixdt(1, 16)  OutScaling=2^-10  DoSatur=off
  Subtract2 : Sum  Inputs=+-
  Switch : Switch  Criteria=u2 > Threshold
  Terminator : Terminator
  Terminator1 : Terminator
  SohOut : Outport
  wires:
  Divide2/1 -> Saturation Dynamic/2
  Chart1/1(SOHWriteResult) -> Terminator/1
  Constant2/1 -> Saturation Dynamic/3
  Constant4/1 -> Divide3/2
  SOC_LeftCap2/1 -> Switch/1, Relational Operator/1
  Divide3/1 -> Divide2/2
  Saturation Dynamic/1 -> Chart1/1(CalcSOH)
  Chart1/2(SohOut) -> SohOut/1
  SOHIn/1 -> [SOHIn], Divide4/3
  Subtract2/1 -> Divide3/1
  Constant1/1 -> Saturation Dynamic/1
  SOC_LeftCap0/1 -> Divide/1
  WOCalibAh/1 -> Divide4/1
  Constant7/1 -> Divide1/2
  Divide1/1 -> Divide/2
  Constant31/1 -> Divide1/1
  Divide/1 -> Relational Operator/2, Subtract2/1
  Relational Operator/1 -> Switch/2
  Constant8/1 -> Switch/3
  Switch/1 -> Subtract2/2
  Constant9/1 -> Divide4/2
  Divide4/1 -> Divide2/1
  [SOHIn] -> Chart1/5(EEEPSOH)
  S-Function1/1 -> Terminator1/1
  Constant10/1 -> S-Function1/2
  DchgPower1/1 -> S-Function1/1
  Constant3/1 -> Chart1/2(MaxDiff)
  Constant6/1 -> Chart1/3(MaxCal)
  Constant5/1 -> Chart1/4(MaxCal1)

== system Udan_SOC/SOC_Calculate/UdanSOCCalcn/CalcDchgSOH/Subsystem1 ==
  HighIndex : Inport
  LowIndex : Inport  Port=2
  DefaultValue : Inport  Port=3
  Constant1 : Constant  Value=0  OutDataTypeStr=uint8
  Constant2 : Constant  Value=0  OutDataTypeStr=uint8
  Logical Operator : Logic  AllPortsSameDT=off  OutDataTypeStr=boolean
  Logical Operator1 : Logic  Operator=NOT  AllPortsSameDT=off  OutDataTypeStr=boolean
  Relational Operator : RelationalOperator  Operator===  OutDataTypeStr=boolean  RndMeth=Simplest
  Relational Operator1 : RelationalOperator  Operator===  OutDataTypeStr=boolean  RndMeth=Simplest
  S-Function : S-Function  FunctionName=sfn_NVMRead  SFunctionDeploymentMode=off  EnableBusSupport=off
  S-Function1 : S-Function  FunctionName=sfn_NVMRead  SFunctionDeploymentMode=off  EnableBusSupport=off
  Subsystem : Subsystem
  Switch : Switch  Criteria=u2 > Threshold
  EeepRead32 : Outport
  wires:
  DefaultValue/1 -> Switch/1
  [ReadLowOk] -> Logical Operator/1
  S-Function/2 -> Subsystem/1(HighIndex)
  S-Function/1 -> Relational Operator/1
  S-Function1/2 -> Subsystem/2(LowIndex)
  HighIndex/1 -> S-Function/1
  Constant1/1 -> Relational Operator/2
  Constant2/1 -> Relational Operator1/2
  LowIndex/1 -> S-Function1/1
  Relational Operator/1 -> Logical Operator/2
  Logical Operator/1 -> Logical Operator1/1, Subsystem/Enable
  Relational Operator1/1 -> [ReadLowOk]
  S-Function1/1 -> Relational Operator1/1
  Subsystem/1(soc) -> Switch/3
  Logical Operator1/1 -> Switch/2
  Switch/1 -> EeepRead32/1

== system Udan_SOC/SOC_Calculate/UdanSOCCalcn/CalcnLeftChargeTime/CalcLeftTime ==
  DLeftCap : Inport
  LowTemp : Inport  Port=2
  PackCur : Inport  Port=3
  TotalCap : Inport  Port=4
  HighTemp : Inport  Port=5
  Enable : EnablePort
  1-D Lookup Table : Lookup_n-D  NumberOfTableDimensions=1  BreakpointsForDimension1=[-5:5]  Table=tanh([-5:5])  InternalRulePriority=Speed  RndMeth=Simplest  InputSameDT=on
  Bus Selector : BusSelector  OutputSignals=FstDecreaseCur,SndDecreaseCur,TrdDecreaseCur,LstDecreaseCur
  Bus Selector1 : BusSelector  OutputSignals=FstDecreaseCur,SndDecreaseCur,TrdDecreaseCur,LstDecreaseCur
  CalcLeftTime : Stateflow chart  TreatAsAtomicUnit=on
  Constant : Constant  Value=9490  OutDataTypeStr=uint16
  Constant1 : Constant  Value=65535  OutDataTypeStr=uint32
  Constant10 : Constant  Value=SOC_SOCResolution  OutDataTypeStr=uint16
  Constant11 : Constant  Value=SOC_SethTempChgValue  OutDataTypeStr=Bus: SOC_ChgCurrentType
  Constant12 : Constant  Value=SOC_EgthTempChgValue  OutDataTypeStr=Bus: SOC_ChgCurrentType
  Constant13 : Constant  Value=SOC_EgthTempChgValue  OutDataTypeStr=Bus: SOC_ChgCurrentType
  Constant14 : Constant  Value=SOC_FstTempChgValue  OutDataTypeStr=Bus: SOC_ChgCurrentType
  Constant15 : Constant  Value=SOC_SndTempChgValue  OutDataTypeStr=Bus: SOC_ChgCurrentType
  Constant16 : Constant  Value=SOC_TrdTempChgValue  OutDataTypeStr=Bus: SOC_ChgCurrentType
  Constant17 : Constant  Value=SOC_FthTempChgValue  OutDataTypeStr=Bus: SOC_ChgCurrentType
  Constant18 : Constant  Value=SOC_FithTempChgValue  OutDataTypeStr=Bus: SOC_ChgCurrentType
  Constant19 : Constant  Value=SOC_SixTempChgValue  OutDataTypeStr=Bus: SOC_ChgCurrentType
  Constant2 : Constant  Value=65535  OutDataTypeStr=uint32
  Constant3 : Constant  Value=SOC_SethTempChgValue  OutDataTypeStr=Bus: SOC_ChgCurrentType
  Constant4 : Constant  Value=SOC_FstTempChgValue  OutDataTypeStr=Bus: SOC_ChgCurrentType
  Constant5 : Constant  Value=SOC_SndTempChgValue  OutDataTypeStr=Bus: SOC_ChgCurrentType
  Constant6 : Constant  Value=SOC_TrdTempChgValue  OutDataTypeStr=Bus: SOC_ChgCurrentType
  Constant7 : Constant  Value=SOC_FthTempChgValue  OutDataTypeStr=Bus: SOC_ChgCurrentType
  Constant8 : Constant  Value=SOC_FithTempChgValue  OutDataTypeStr=Bus: SOC_ChgCurrentType
  Constant9 : Constant  Value=SOC_SixTempChgValue  OutDataTypeStr=Bus: SOC_ChgCurrentType
  Divide : Product  Inputs=*/*  OutDataTypeStr=uint32
  Divide1 : Product  Inputs=*/*  OutDataTypeStr=uint32
  Divide2 : Product  Inputs=*/*  OutDataTypeStr=uint32
  MinMax{,1..3} (4 alike) : MinMax  Inputs=2
  SelectChgCurrent : Stateflow chart  TreatAsAtomicUnit=on
  SelectChgCurrent1 : Stateflow chart  TreatAsAtomicUnit=on
  Terminator : Terminator
  Terminator1 : Terminator
  LeftChargeTime : Outport
  PackCurOk : Outport  Port=2
  wires:
  Constant/1 -> Divide/3
  Constant10/1 -> Divide1/3, Divide2/2, Divide2/3, Divide1/2, Divide/2
  LowTemp/1 -> SelectChgCurrent/1(BatTemp)
  Constant4/1 -> SelectChgCurrent/2(FstChgCur)
  Constant5/1 -> SelectChgCurrent/3(SndChgCur)
  Constant6/1 -> SelectChgCurrent/4(TrdChgCur)
  Constant7/1 -> SelectChgCurrent/5(FthChgCur)
  Constant8/1 -> SelectChgCurrent/6(FithChgCur)
  Constant9/1 -> SelectChgCurrent/7(SixChgCur)
  Constant11/1 -> SelectChgCurrent/8(SevenChgCur)
  Constant12/1 -> SelectChgCurrent/9(EgthTempChgValue)
  SelectChgCurrent/1(ChgCurOut) -> Bus Selector/1
  DLeftCap/1 -> CalcLeftTime/1(DleftCap)  "LastDCapWODelay"
  TotalCap/1 -> CalcLeftTime/3(NominalCap), Divide2/1, Divide1/1, Divide/1
  Divide/1 -> CalcLeftTime/4(FstDecPnt)
  Constant1/1 -> CalcLeftTime/5(SndDecPnt)
  Constant2/1 -> CalcLeftTime/6(TrdDecPnt)
  CalcLeftTime/1(TimeOut) -> LeftChargeTime/1  "TimeOut"
  PackCur/1 -> CalcLeftTime/2(PackCur)
  CalcLeftTime/2(result) -> PackCurOk/1
  Constant13/1 -> SelectChgCurrent1/9(EgthTempChgValue)
  Constant16/1 -> SelectChgCurrent1/4(TrdChgCur)
  Constant3/1 -> SelectChgCurrent1/8(SevenChgCur)
  Constant18/1 -> SelectChgCurrent1/6(FithChgCur)
  Constant17/1 -> SelectChgCurrent1/5(FthChgCur)
  HighTemp/1 -> SelectChgCurrent1/1(BatTemp)
  Constant19/1 -> SelectChgCurrent1/7(SixChgCur)
  Constant15/1 -> SelectChgCurrent1/3(SndChgCur)
  Constant14/1 -> SelectChgCurrent1/2(FstChgCur)
  Bus Selector1/1 -> [HighTemp_FstDecCur]  "<FstDecreaseCur>"
  SelectChgCurrent1/1(ChgCurOut) -> Bus Selector1/1
  Bus Selector1/3 -> [HighTemp_TrdDecCur]  "<TrdDecreaseCur>"
  Bus Selector1/2 -> [HighTemp_SndDecCur]  "<SndDecreaseCur>"
  Bus Selector1/4 -> [LstTemp_LastDecCur]  "<LstDecreaseCur>"
  MinMax/1 -> CalcLeftTime/7(Cur1)  "cur1"
  [HighTemp_FstDecCur] -> MinMax/2
  Bus Selector/1 -> MinMax/1  "<FstDecreaseCur>"
  MinMax1/1 -> CalcLeftTime/8(Cur2)
  [HighTemp_SndDecCur] -> MinMax1/2
  MinMax2/1 -> CalcLeftTime/9(Cur3)
  [HighTemp_TrdDecCur] -> MinMax2/2
  MinMax3/1 -> CalcLeftTime/10(Cur4)
  [LstTemp_LastDecCur] -> MinMax3/2
  Bus Selector/2 -> MinMax1/1  "<SndDecreaseCur>"
  Bus Selector/3 -> MinMax2/1  "<TrdDecreaseCur>"
  Bus Selector/4 -> MinMax3/1  "<LstDecreaseCur>"
  Divide1/1 -> Terminator/1
  Divide2/1 -> Terminator1/1
